simulink model "test_motion_law_block"  (R2021b)
settings: Solver=FixedStepAuto  StartTime=0.0  StopTime=50  FixedStep=Ts  RelTol=1e-3
values from neighbouring files (symbols this model uses):
  Ts = 1e-3    (= 0.001)    [load_data.m]    (also in run_test_motion_law_block.m; run_test_motion_logic.m; run_test_switch_sensor.m; testWegMotionLaw.m)
libraries: LiftMotionControlLibrary x1
settings Model: Creator=manue  LastModifiedBy=manue
settings DataIOCC: SaveFormat=StructureWithTime

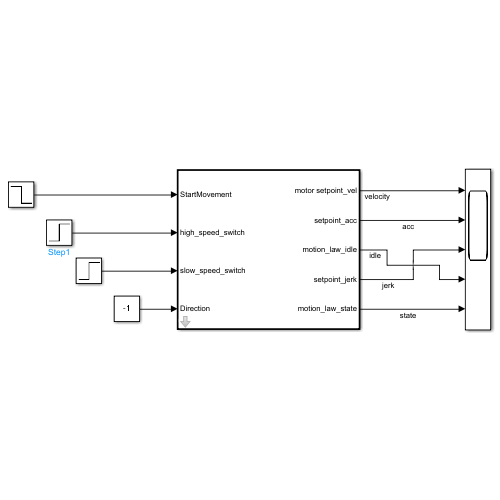
[thumbnail: Simulink's stored preview of the top-level diagram]
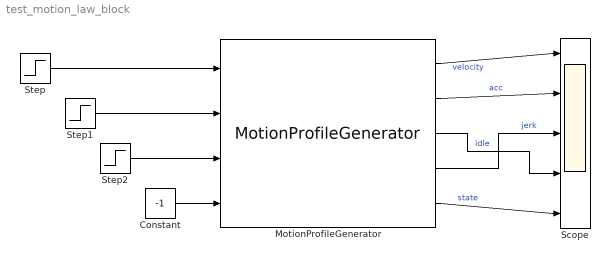
== system test_motion_law_block ==
  Constant : Constant  Value=-1
  MotionProfileGenerator : LiftMotionControlLibrary/MotionProfileGenerator  Ts=Ts  gearbox=gearbox  Rp=Rp  HighSpeed=HighSpeed  LowSpeed=LowSpeed  PercentAccFactor=PercentAccFactor  AccelInitialJerk=AccelInitialJerk  Acceleration=Acceleration  AccelEndJerk=AccelEndJerk  DecelInitialJerk=DecelInitialJerk  Deceleration=Deceleration  DecelEndJerk=DecelEndJerk  StopDeceleration=StopDeceleration
  Scope : Scope  NumInputPorts=5
  Step : Step  Before=1  After=0  SampleTime=0
  Step1 : Step  Time=30  SampleTime=0
  Step2 : Step  Time=35  SampleTime=0
  wires:
  Step/1 -> MotionProfileGenerator/1
  Step1/1 -> MotionProfileGenerator/2
  Step2/1 -> MotionProfileGenerator/3
  Constant/1 -> MotionProfileGenerator/4
  MotionProfileGenerator/1 -> Scope/1  "velocity"
  MotionProfileGenerator/2 -> Scope/2  "acc"
  MotionProfileGenerator/4 -> Scope/3  "jerk"
  MotionProfileGenerator/3 -> Scope/4  "idle"
  MotionProfileGenerator/5 -> Scope/5  "state"
